simulink model "quadcopter_eselu"  (R2016b)
settings: Solver=ode3  StartTime=0.0  StopTime=30  FixedStep=0.001  MaxStep=0.004  RelTol=1e-3
PreLoadFcn:
  | init
settings Model: Creator=ADAM  LastModifiedBy=consti
settings SolverCC: ExtrapolationOrder=1
settings DataIOCC: MaxDataPoints=1  SaveFormat=Structure  SignalLoggingSaveFormat=ModelDataLogs  SaveOutput=off  SignalLogging=off  DSMLogging=off  SaveTime=off  OutputSaveName=model_out  SignalLoggingName=model_out
settings OptimizationCC: ExpressionDepthLimit=2147483647  LifeSpan=inf  SimCompilerOptimization=on
settings DebuggingCC: UnderspecifiedInitializationDetection=Classic  MergeDetectMultiDrivingBlocksExec=none  InheritedTsInSrcMsg=none  MultiTaskDSMMsg=warning  MultiTaskCondExecSysMsg=none  UnconnectedInputMsg=none  UnconnectedOutputMsg=none  UnconnectedLineMsg=none  StateNameClashWarn=warning  SFUnexpectedBacktrackingDiag=warning  SFNoUnconditionalDefaultTransitionDiag=warning  SFExecutionAtInitializationDiag=none
settings HardwareCC: ProdBitPerPointer=32  ProdBitPerSizeT=32  ProdBitPerPtrDiffT=32  ProdLargestAtomicFloat=None  ProdWordSize=32  ProdHWDeviceType=Generic->32-bit x86 compatible
settings ModelReferenceCC: PropagateSignalLabelsOutOfModel=off
settings CodeAppCC: MaxIdLength=95
settings GRTTargetCC: TargetLangStandard=C89/C90 (ANSI)  GeneratePreprocessorConditionals=Disable all
settings ConfigComp: CovMetricSettings=dw  CovHtmlReporting=on  CovSaveCumulativeToWorkspaceVar=on  CovSaveSingleToWorkspaceVar=on  CovExternalEMLEnable=off  CovSFcnEnable=off

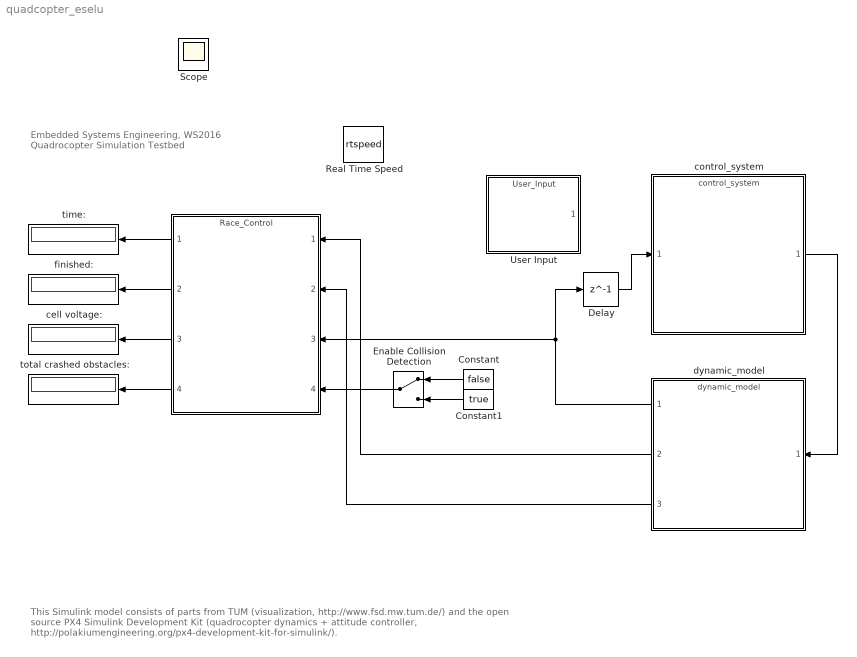
== system quadcopter_eselu ==
  note: Embedded Systems Engineering, WS2016
      | Quadrocopter Simulation Testbed
  note: This Simulink model consists of parts from TUM (visualization, http://www.fsd.mw.tum.de/) and the open source PX4 Simulink Development Kit (quadrocopter dynamics + attitude controller, http://polakiumengineering.org/px4-development-kit-for-simulink/).
  " " : ModelReference  ModelNameDialog=Race_Control.slx  SimulationMode=Normal  ModelReferenceVersion=1.2428
  Constant : Constant  Value=false
  Constant1 : Constant  Value=true
  Delay : Delay  DelayLength=1
  Enable Collision Detection : ManualSwitch
  Real Time Speed : S-Function  FunctionName=rtspeed  Parameters=speed  SFunctionDeploymentMode=off  EnableBusSupport=off  mask(Simulink Realtime Synchronization){speed=1}
      mask prompts: speed "Simulation Speed (1 = realtime)"
      mask help: Slows down simulation to desired real time speed.
      mask Display:
      | ang=(0:0.0125:1)*2*pi;
      | xp=100*cos(ang);
      | yp=100*sin(ang);
      | plot(-145,-130,155,170,xp,yp,[0 0 70*sqrt(2)/2],[70 0 70*sqrt(2)/2],[-40 40 40 -40 -40],[150 150 120 120 150],[-15 -15],[120 98.5],[15 15],[120 98.5],[100*cos((45+9)/180*pi) 100*cos((45+9)/180*pi)+30 100*cos((45-9)/180*pi)+30 100*cos((45-9)/180*pi)],[100*sin((45+9)/180*pi) 100*sin((45+9)/180*pi)+30 100*sin((45-9)/180*pi)+30 100*sin((45-9)/180*pi)]);
  User Input : ModelReference  ModelNameDialog=User_Input.slx  SimulationMode=Normal  ModelReferenceVersion=1.2320
  cell voltage: : Display
  control_system : ModelReference  ModelNameDialog=control_system  SimulationMode=Normal  ModelReferenceVersion=1.2836
  dynamic_model : ModelReference  ModelNameDialog=dynamic_model  SimulationMode=Normal  ModelReferenceVersion=1.2326
  finished: : Display
  time: : Display
  total crashed obstacles: : Display
  Scope : Scope
  wires:
  dynamic_model/2 -> " "/1
  dynamic_model/3 -> " "/2
  control_system/1 -> dynamic_model/1
  dynamic_model/1 -> " "/3, Delay/1
  Delay/1 -> control_system/1
  " "/1 -> time:/1
  " "/2 -> finished:/1
  " "/3 -> cell voltage:/1
  Enable Collision Detection/1 -> " "/4
  Constant/1 -> Enable Collision Detection/1
  Constant1/1 -> Enable Collision Detection/2
  " "/4 -> total crashed obstacles:/1
